simulink model "Phi"  (R2024a)
settings: Solver=VariableStepAuto  StartTime=0.0  StopTime=7  RelTol=1e-3
values from neighbouring files (symbols this model uses):
  K = 0.38    [RunCphi.m]    (also in RunCrho.m = 0.07; RunGphi.m; RunGrho.m = 0.07; RunPhi.m)
  Kp = 1    [RunCphi.m]    (also in RunCrho.m = 28; RunPhi.m = 20; RunRho.m = 28; Runmotor_control.m = 2.8)
  sigma = 8.5    [RunCphi.m]    (also in RunCrho.m = 11; RunGphi.m; RunGrho.m = 11; RunPhi.m)
libraries: simulink x1, slpidlib x1
settings Model: Creator=sansh  LastModifiedBy=liama
settings SolverCC: AlgebraicLoopSolver=TrustRegion
settings DataIOCC: ReturnWorkspaceOutputs=off
settings DebuggingCC: UnconnectedInputMsg=warning  UnconnectedOutputMsg=warning  UnconnectedLineMsg=warning  ArithmeticOperatorsInVariantConditions=warning
settings ModelReferenceCC: EnableRefExpFcnMdlSchedulingChecks=on
settings SFSimCC: SimUseLocalCustomCode=off  CustomCodeUndefinedFunction=UseInterfaceOnly
settings RTWCC: RTWUseLocalCustomCode=off  GPUComputeCapability=3.5
settings CodeAppCC: StateflowObjectComments=on

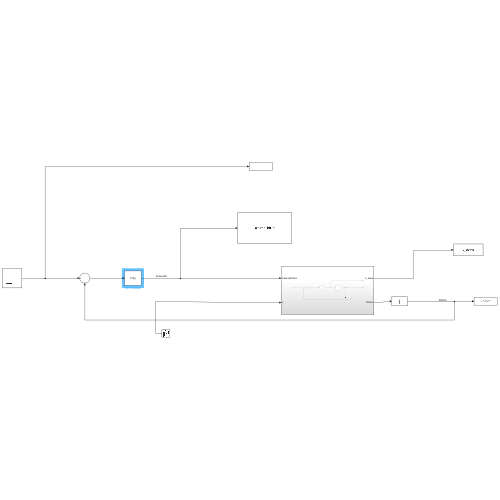
[thumbnail: Simulink's stored preview of the top-level diagram]
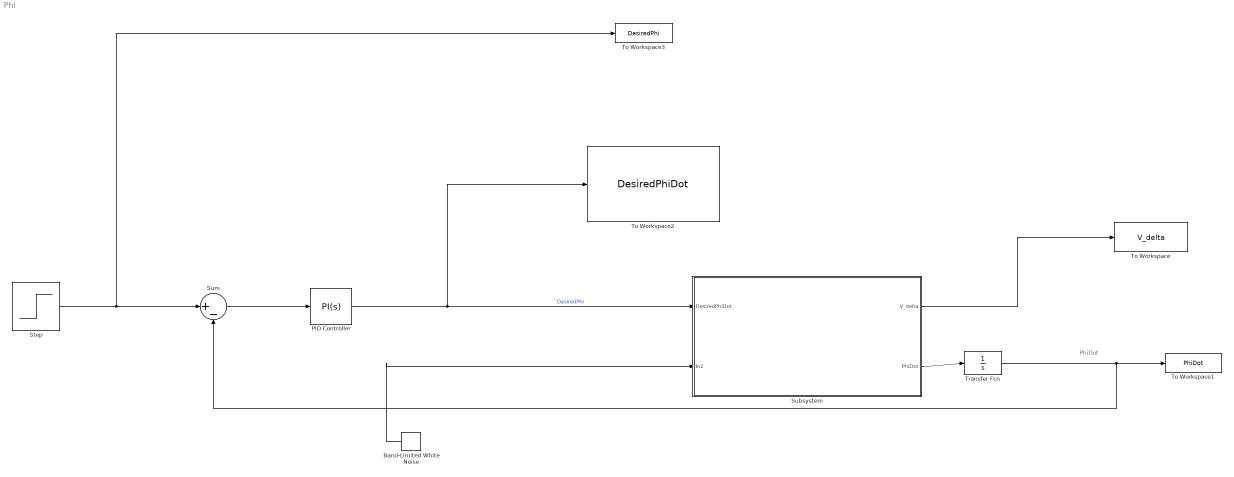
== system Phi ==
  note: PhiDot
  Band-Limited White Noise : simulink/Sources/Band-Limited White Noise  Cov=[0.0005]  Ts=0.1  seed=[23341]
  PID Controller : slpidlib/PID Controller  Controller=PI  Form=Parallel  TimeDomain=Continuous-time  UseExternalTs=off  SampleTime=-1  IntegratorMethod=Forward Euler  FilterMethod=Forward Euler  ControllerParametersSource=internal  P=27.5212039531514  I=139.174517974539  UseKiTs=off  D=1.77297218610117  UseExternalDerivativeSource=off  N=474.788175851999  UseFilter=on  TunerSelectOption=Transfer Function Based (PID Tuner App)  InitialConditionSource=internal  InitialConditionForIntegrator=0  InitialConditionForFilter=0  DifferentiatorICPrevScaledInput=0  ExternalReset=none  TrackingMode=off  Kt=1  LimitOutput=off  SatLimitsSource=internal  UpperSaturationLimit=inf  LowerSaturationLimit=-inf  LinearizeAsGain=on  AntiWindupMode=none  Kb=1  LimitIntegrator=off  UpperIntegratorSaturationLimit=inf  LowerIntegratorSaturationLimit=-inf  POutMin=[]  POutMax=[]  IOutMin=[]  IOutMax=[]  DOutMin=[]  DOutMax=[]  NOutMin=[]  NOutMax=[]  SumOutMin=[]  SumOutMax=[]  SaturationOutMin=[]  SaturationOutMax=[]  PParamMin=[]  PParamMax=[]  IParamMin=[]  IParamMax=[]  DParamMin=[]  DParamMax=[]  NParamMin=[]  NParamMax=[]  KbParamMin=[]  KbParamMax=[]  KtParamMin=[]  KtParamMax=[]  KbOutMin=[]  KbOutMax=[]  KtOutMin=[]  KtOutMax=[]  IntegratorOutMin=[]  IntegratorOutMax=[]  FilterOutMin=[]  FilterOutMax=[]  SumI1OutMin=[]  SumI1OutMax=[]  SumI2OutMin=[]  SumI2OutMax=[]  SumI3OutMin=[]  SumI3OutMax=[]  SumI4OutMin=[]  SumI4OutMax=[]  SumDOutMin=[]  SumDOutMax=[]  DifferentiatorOutMin=[]  DifferentiatorOutMax=[]  FilterDiffOutCoefMin=[]  FilterDiffOutCoefMax=[]  ReciprocalOutMin=[]  ReciprocalOutMax=[]  SumDenOutMin=[]  SumDenOutMax=[]  SumNumOutMin=[]  SumNumOutMax=[]  DivideOutMin=[]  DivideOutMax=[]  UdiffTsProdOutMin=[]  UdiffTsProdOutMax=[]  NTsProdOutMin=[]  NTsProdOutMax=[]  UintegralTsProdOutMin=[]  UintegralTsProdOutMax=[]  UngainTsProdOutMin=[]  UngainTsProdOutMax=[]  ClampingZeroOutDataTypeStr=Inherit: Inherit via back propagation  ClampingZeroOutMin=[]  ClampingZeroOutMax=[]  FilterDenConstantOutDataTypeStr=Inherit: Inherit via back propagation  FilterDenConstantOutMin=[]  FilterDenConstantOutMax=[]  PCopyOutDataTypeStr=Inherit: Inherit via back propagation  PCopyOutMin=[]  PCopyOutMax=[]  NCopyOutDataTypeStr=Inherit: Inherit via back propagation  NCopyOutMin=[]  NCopyOutMax=[]  IntegratorContinuousStateAttributes=''  IntegratorStateMustResolveToSignalObject=off  IntegratorRTWStateStorageClass=Auto  FilterContinuousStateAttributes=''  FilterStateMustResolveToSignalObject=off  FilterRTWStateStorageClass=Auto  ParallelPVariant=InternalParameters  IdealPVariant=Disabled  IVariant=InternalParameters  DVariant=Disabled  IntegratorVariant=Continuous  SatVariant=Disabled  AWVariant=Passthrough  PCopyVariant=Disabled  TRVariant=Disabled  FdbkBlocksVariant=Forward  IdealPFdbkVariant=Disabled  SatFdbkVariant=Disabled  DerivativeFilterVariant=Disabled  NVariant=Disabled  NCopyVariant=Disabled_SignalSpec  FilterICVariant=Disabled  IntegratorICVariant=InternalICs  ExternalResetVariant=Disabled  TRSumVariant=Passthrough  SumFdbkVariant=Disabled  SumVariant=Sum_PI  TsampFilterVariant=InternalTs  TsampNgainVariant=Passthrough  TsampIntegralVariant=Disabled_SignalSpec  ExternalSaturationOutDataTypeStr=Inherit: Same as second input  DerivativeSourceVariant=Disabled
  Step : Step  Time=2  SampleTime=0
  Subsystem : Subsystem
  Sum : Sum  Inputs=|+-
  To Workspace : ToWorkspace  VariableName=V_delta  SaveFormat=Timeseries  SampleTime=-1
  To Workspace1 : ToWorkspace  VariableName=PhiDot  SaveFormat=Timeseries  SampleTime=-1
  To Workspace2 : ToWorkspace  VariableName=DesiredPhiDot  SaveFormat=Timeseries  SampleTime=-1
  To Workspace3 : ToWorkspace  VariableName=DesiredPhi  SaveFormat=Timeseries  SampleTime=-1
  Transfer Fcn : TransferFcn  Denominator=[1 0]
  wires:
  PID Controller/1 -> To Workspace2/1, Subsystem/1(DesiredPhiDot)  "DesiredPhi"
  Band-Limited White Noise/1 -> Subsystem/2(In2)
  Subsystem/1(V_delta) -> To Workspace/1
  Sum/1 -> PID Controller/1
  Subsystem/2(PhiDot) -> Transfer Fcn/1
  Transfer Fcn/1 -> To Workspace1/1, Sum/2
  Step/1 -> To Workspace3/1, Sum/1

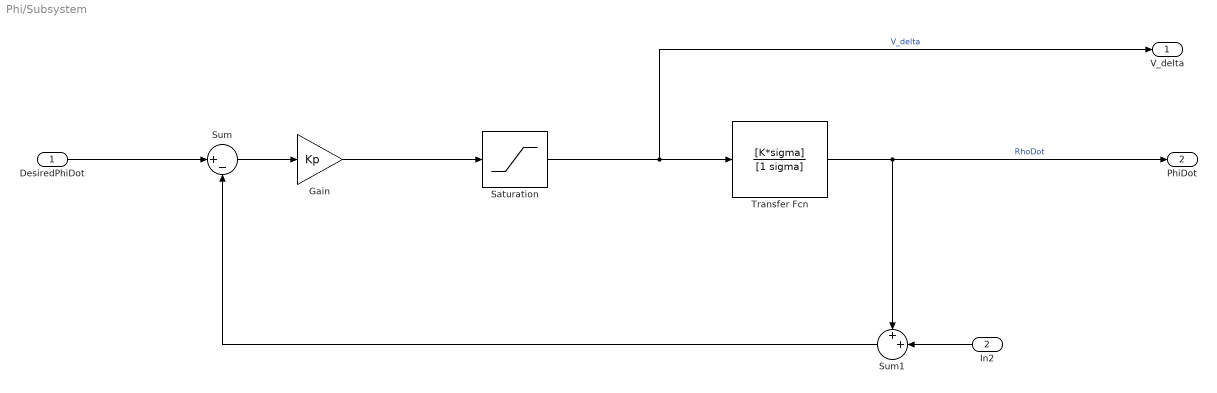
== system Phi/Subsystem ==
  DesiredPhiDot : Inport
  In2 : Inport  Port=2
  Gain : Gain  Gain=Kp
  Saturation : Saturate  UpperLimit=16.8  LowerLimit=-16.8
  Sum : Sum  Inputs=|+-
  Sum1 : Sum  Inputs=++|
  Transfer Fcn : TransferFcn  Numerator=[K*sigma]  Denominator=[1 sigma]
  V_delta : Outport
  PhiDot : Outport  Port=2
  wires:
  Sum1/1 -> Sum/2
  Transfer Fcn/1 -> PhiDot/1, Sum1/1  "RhoDot"
  Sum/1 -> Gain/1
  In2/1 -> Sum1/2
  Saturation/1 -> V_delta/1, Transfer Fcn/1  "V_delta"
  Gain/1 -> Saturation/1
  DesiredPhiDot/1 -> Sum/1
